simulink model "motor1"  (R2021b)
settings: Solver=VariableStepAuto  StartTime=0.0  StopTime=10.0  RelTol=1e-3
settings Model: Creator=marbl  LastModifiedBy=marbl
settings DebuggingCC: UnconnectedInputMsg=none  UnconnectedOutputMsg=none  UnconnectedLineMsg=none
settings ModelReferenceCC: EnableRefExpFcnMdlSchedulingChecks=off
settings RTWCC: GPUComputeCapability=5.0  DLArmComputeVersion=20.02.1

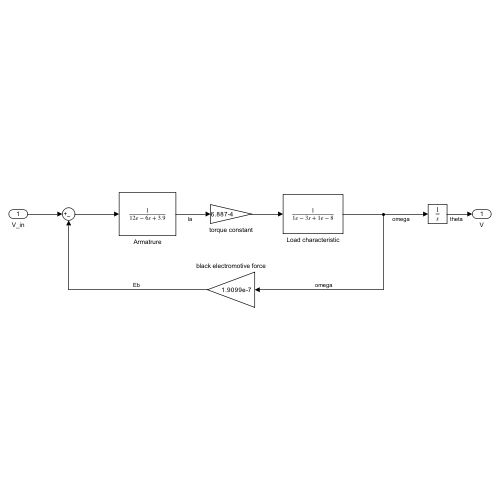
[thumbnail: Simulink's stored preview of the top-level diagram]
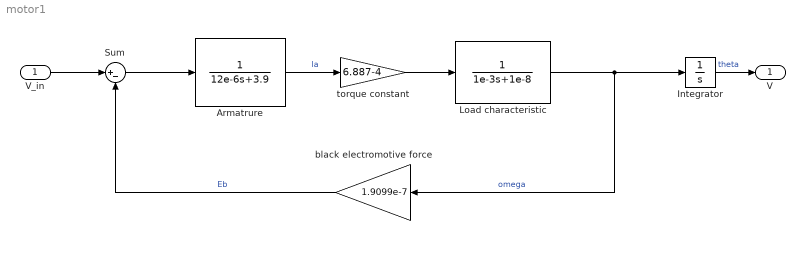
== system motor1 ==
  V_in : Inport
  Armatrure : TransferFcn  Denominator="[12e-6  3.9]"
  Integrator : Integrator
  Load characteristic : TransferFcn  Denominator=[1e-3 1e-8]
  Sum : Sum  Inputs=|+-
  black electromotive force : Gain  Gain=1.9099e-7
  torque constant : Gain  Gain=6.887-4
  V : Outport
  wires:
  V_in/1 -> Sum/1
  Armatrure/1 -> torque constant/1  "la"
  Sum/1 -> Armatrure/1
  torque constant/1 -> Load characteristic/1
  Load characteristic/1 -> Integrator/1, black electromotive force/1  "omega"
  black electromotive force/1 -> Sum/2  "Eb"
  Integrator/1 -> V/1  "theta"
